simulink model "controller_lat"  (R2017b)
settings: Solver=VariableStepAuto  StartTime=0.0  StopTime=10  RelTol=1e-3
values from neighbouring files (symbols this model uses):
  alphax = opreport.Outputs(13).y    [controller_lat_design.m]    (also in lat_gain20190526.mat = 0.0698131700798)
  CSim_phi = 1    [controller_lat_design.m]    (also in lat_gain20190526.mat)
  CSim_r = 0    [controller_lat_design.m]    (also in lat_gain20190526.mat)
  K_ARI = -0.1    [controller_lat_design.m]    (also in lat_gain20190526.mat = 0.298094672282)
  KF_phi = 0    [controller_lat_design.m]    (also in lat_gain20190526.mat = -1.34430735643)
  KI_phi = 0    [controller_lat_design.m]    (also in lat_gain20190526.mat = 1.99482743972)
  KP_p = 1    [controller_lat_design.m]    (also in lat_gain20190526.mat = 0.210525781723)
  KP_p2 = 1    [controller_lat_design.m]    (also in lat_gain20190526.mat = 0.786351487124)
  KP_phi = 1    [controller_lat_design.m]    (also in lat_gain20190526.mat = 1.78064492258)
  KP_r = 0.1    [controller_lat_design.m]    (also in lat_gain20190526.mat = 0.189713272044)
  Tau_DA = 0.05    [controller_lat_design.m]    (also in lat_gain20190526.mat)
  Tau_DR = 0.05    [controller_lat_design.m]    (also in lat_gain20190526.mat)
  tauw_r = 5    [controller_lat_design.m]    (also in lat_gain20190526.mat)
undefined symbols (not defined in the file or in its folder): Actuators, Linmod
settings Model: Creator=zht  LastModifiedBy=zht

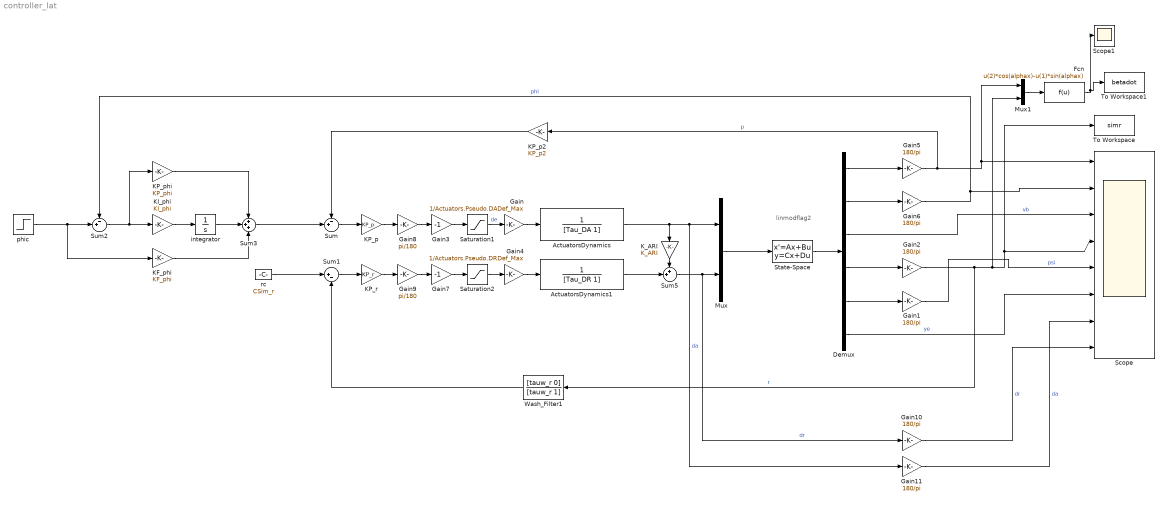
== system controller_lat ==
  note: linmodflag2
  ActuatorsDynamics : TransferFcn  Denominator=[Tau_DA 1]
  ActuatorsDynamics1 : TransferFcn  Denominator=[Tau_DR 1]
  Demux : Demux  Outputs=6
  Fcn : Fcn  Expr=u(2)*cos(alphax)-u(1)*sin(alphax)
  Gain : Gain  Gain=1/Actuators.Pseudo.DADef_Max
  Gain{1..2,5..6,10..11} (6 alike) : Gain  Gain=180/pi
  Gain3 : Gain  Gain=-1
  Gain4 : Gain  Gain=1/Actuators.Pseudo.DRDef_Max
  Gain7 : Gain  Gain=-1
  Gain8 : Gain  Gain=pi/180
  Gain9 : Gain  Gain=pi/180
  KF_phi : Gain  Gain=KF_phi
  KI_phi : Gain  Gain=KI_phi
  KP_p : Gain  Gain=KP_p
  KP_p2 : Gain  Gain=KP_p2
  KP_phi : Gain  Gain=KP_phi
  KP_r : Gain  Gain=KP_r
  K_ARI : Gain  Gain=K_ARI
  Mux : Mux  Inputs=2
  Mux1 : Mux  Inputs=2
  Saturation1 : Saturate  UpperLimit=Actuators.Pseudo.DADef_Max  LowerLimit=-Actuators.Pseudo.DADef_Max
  Saturation2 : Saturate  UpperLimit=Actuators.Pseudo.DRDef_Max  LowerLimit=-Actuators.Pseudo.DRDef_Max
  Scope : Scope  NumInputPorts=8
  Scope1 : Scope
  State-Space : StateSpace  A=Linmod.Lat_6.A  B=Linmod.Lat_6.B  C=Linmod.Lat_6.C  D=Linmod.Lat_6.D  InitialCondition=0  ContinuousStateAttributes={'p','Phi','vb','r','psi','ye'}
  Sum : Sum  Inputs=-+|
  Sum1 : Sum  Inputs=|+-
  Sum2 : Sum  Inputs=-+|
  Sum3 : Sum  Inputs=+++
  Sum5 : Sum  Inputs=++|
  To Workspace : ToWorkspace  VariableName=simr  SaveFormat=Timeseries  SampleTime=-1
  To Workspace1 : ToWorkspace  VariableName=betadot  SaveFormat=Timeseries  SampleTime=-1
  Wash_Filter1 : TransferFcn  Numerator=[tauw_r 0]  Denominator=[tauw_r 1]
  integrator : Integrator
  phic : Step  Time=0  After=CSim_phi  SampleTime=0
  rc : Constant  Value=CSim_r
  wires:
  Mux/1 -> State-Space/1
  rc/1 -> Sum1/1
  State-Space/1 -> Demux/1
  Demux/2 -> Gain6/1
  Demux/4 -> Gain2/1
  Demux/5 -> Gain1/1
  Demux/1 -> Gain5/1
  Demux/3 -> Scope/3  "vb"
  Gain2/1 -> Wash_Filter1/1, Mux1/2, To Workspace/1, Scope/4  "r"
  Gain/1 -> ActuatorsDynamics/1
  Sum/1 -> KP_p/1
  Sum3/1 -> Sum/2
  Sum2/1 -> KP_phi/1, KI_phi/1
  Saturation1/1 -> Gain/1  "de"
  Gain3/1 -> Saturation1/1
  ActuatorsDynamics/1 -> K_ARI/1, Gain11/1, Mux/1  "da"
  phic/1 -> Sum2/2, KF_phi/1
  KP_p/1 -> Gain8/1
  integrator/1 -> Sum3/2
  KF_phi/1 -> Sum3/3
  KP_phi/1 -> Sum3/1
  KI_phi/1 -> integrator/1
  Sum5/1 -> Gain10/1, Mux/2  "dr"
  Gain4/1 -> ActuatorsDynamics1/1
  Saturation2/1 -> Gain4/1
  Demux/6 -> Scope/6  "ye"
  Gain5/1 -> Mux1/1, Scope/1, KP_p2/1  "p"
  Gain6/1 -> Sum2/1, Scope/2  "phi"
  Gain1/1 -> Scope/5  "psi"
  KP_p2/1 -> Sum/1
  Sum1/1 -> KP_r/1
  Gain7/1 -> Saturation2/1
  KP_r/1 -> Gain9/1
  Mux1/1 -> Fcn/1
  Fcn/1 -> To Workspace1/1, Scope1/1
  Wash_Filter1/1 -> Sum1/2
  ActuatorsDynamics1/1 -> Sum5/2
  K_ARI/1 -> Sum5/1
  Gain8/1 -> Gain3/1
  Gain9/1 -> Gain7/1
  Gain10/1 -> Scope/8  "dr"
  Gain11/1 -> Scope/7  "da"
